simulink model "PT1_testbench"  (R2025b)
settings: Solver=VariableStepAuto  StartTime=0.0  StopTime=10.0  RelTol=1e-3
PreLoadFcn:
  | T=1;
  | Kp=1;
model workspace (MAT data in the model file):
  Kp = 0.5
  T = 2
settings Model: Creator=danieltchoudovski  LastModifiedBy=danieltchoudovski

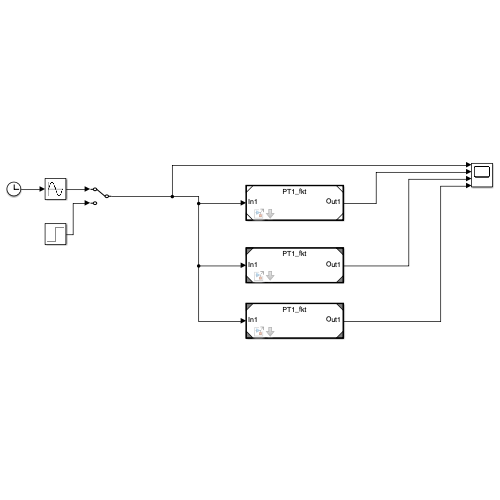
[thumbnail: Simulink's stored preview of the top-level diagram]
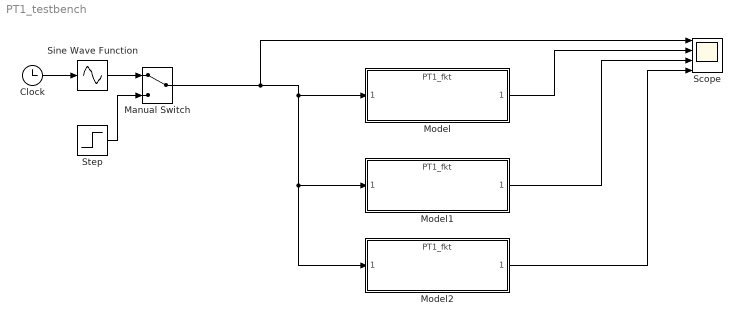
== system PT1_testbench ==
  Clock : Clock
  Manual Switch : ManualSwitch
  Model : ModelReference  ModelNameDialog=PT1_fkt.slx  UsingDefaultArgumentValue=0,0  SimulationMode=Normal  ModelReferenceVersion=1.12  mask{Kp=0.5, T=2}
  Model1 : ModelReference  ModelNameDialog=PT1_fkt  UsingDefaultArgumentValue=0,0  SimulationMode=Normal  ModelReferenceVersion=1.12  mask{Kp=2, T=2}
  Model2 : ModelReference  ModelNameDialog=PT1_fkt  UsingDefaultArgumentValue=0,0  SimulationMode=Normal  ModelReferenceVersion=1.12  mask{Kp=3, T=0.5}
  Scope : Scope  NumInputPorts=4
      settings: ActiveDisplayYMinimum=-2.65050221069472  ActiveDisplayYMaximum=2.8075013137412528
  Sine Wave Function : Sin  TimeSource=Use external signal  SampleTime=0
  Step : Step  SampleTime=0
  wires:
  Clock/1 -> Sine Wave Function/1
  Manual Switch/1 -> Model/1, Model2/1, Model1/1, Scope/1
  Model/1 -> Scope/2
  Model1/1 -> Scope/3
  Model2/1 -> Scope/4
  Step/1 -> Manual Switch/2
  Sine Wave Function/1 -> Manual Switch/1
